simulink model "ev4 (1)"  (R2024a)
settings: Solver=VariableStepAuto  StartTime=0.0  StopTime=601  MaxStep=0.0001  RelTol=1e-3
values from neighbouring files (symbols this model uses):
  a = 1    [evsimcode.m]
  ap = 1.07    [evsimcode.m]
  cd = 0.8    [evsimcode.m]
  ce = 0.9    [evsimcode.m]
  cell_c = 5    [evsimcode.m]
  cell_v = 3.6    [evsimcode.m]
  cr = 0.05    [evsimcode.m]
  cur = data2(:,1)    [evsimcode.m]
  eff = data2(:,5)    [evsimcode.m]
  g = 9.81    [evsimcode.m]
  gr = 9.2    [evsimcode.m]
  lap = 10    [evsimcode.m]
  m = 260    [evsimcode.m]
  me = 0.85    [evsimcode.m]
  ocv = data(:,2)    [evsimcode.m]
  pow = data2(:,2)    [evsimcode.m]
  rho = 1.225    [evsimcode.m]
  rw = 0.2921    [evsimcode.m]
  soc = data(:,1)    [evsimcode.m]
  spd = data2(:,4)    [evsimcode.m]
  te = 0.88    [evsimcode.m]
  theta = 0.6457718232    [evsimcode.m]
  tor = data2(:,2)    [evsimcode.m]
  v = 48    [evsimcode.m]
settings Model: Creator=AXISNIEL  LastModifiedBy=Sai Vivek
settings DebuggingCC: UnconnectedInputMsg=warning  UnconnectedOutputMsg=warning  UnconnectedLineMsg=warning
settings ModelReferenceCC: EnableRefExpFcnMdlSchedulingChecks=on
settings RTWCC: GPUComputeCapability=3.5  DLArmComputeVersion=19.05

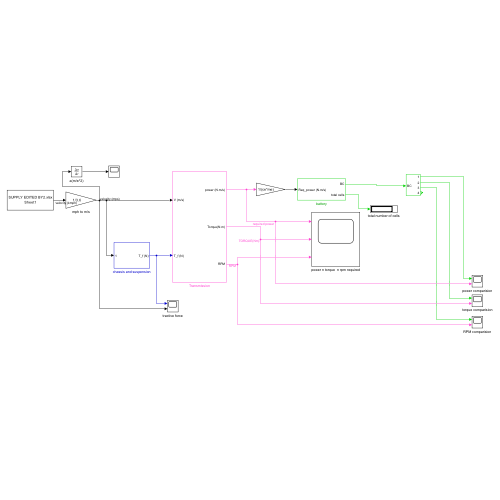
[thumbnail: Simulink's stored preview of the top-level diagram]
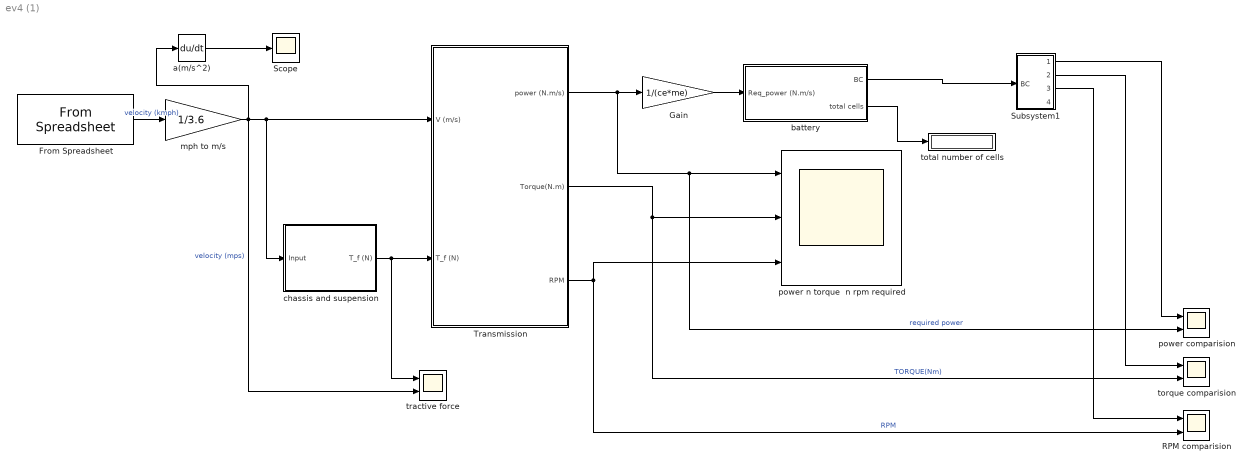
== system ev4 (1) ==
  From Spreadsheet : FromSpreadsheet  FileName=SUPPLY EDITED BY2.xlsx  Range=A1:B601
  Gain : Gain  Gain=1/(ce*me)
  RPM comparision : Scope  NumInputPorts=2
  Scope : Scope
  Subsystem1 : Subsystem
  Transmission : Subsystem
  a(m/s^2) : Derivative
  battery : Subsystem
  chassis and suspension : Subsystem
  mph to m/s : Gain  Gain=1/3.6
  power comparision : Scope  NumInputPorts=2
  power n torque  n rpm required : Scope  NumInputPorts=3
  torque comparision : Scope  NumInputPorts=2
  total number of cells : Display
  tractive force : Scope  NumInputPorts=2
  wires:
  Gain/1 -> battery/1(Req_power (N.m/s))
  Transmission/1(power (N.m/s)) -> Gain/1, power n torque  n rpm required/1, power comparision/2  "required power"
  Transmission/2(Torque(N.m)) -> power n torque  n rpm required/2, torque comparision/2  "TORQUE(Nm)"
  From Spreadsheet/1 -> mph to m/s/1  "velocity (kmph)"
  battery/1(BC) -> Subsystem1/1(BC)
  mph to m/s/1 -> a(m/s^2)/1, chassis and suspension/1(Input), Transmission/1(V (m/s)), tractive force/2  "velocity (mps)"
  Transmission/3(RPM) -> power n torque  n rpm required/3, RPM comparision/2  "RPM"
  chassis and suspension/1(T_f (N)) -> Transmission/2(T_f (N)), tractive force/1
  battery/2(total cells) -> total number of cells/1
  Subsystem1/1(Out1) -> power comparision/1
  Subsystem1/2(Out2) -> torque comparision/1
  Subsystem1/3(Out3) -> RPM comparision/1
  a(m/s^2)/1 -> Scope/1

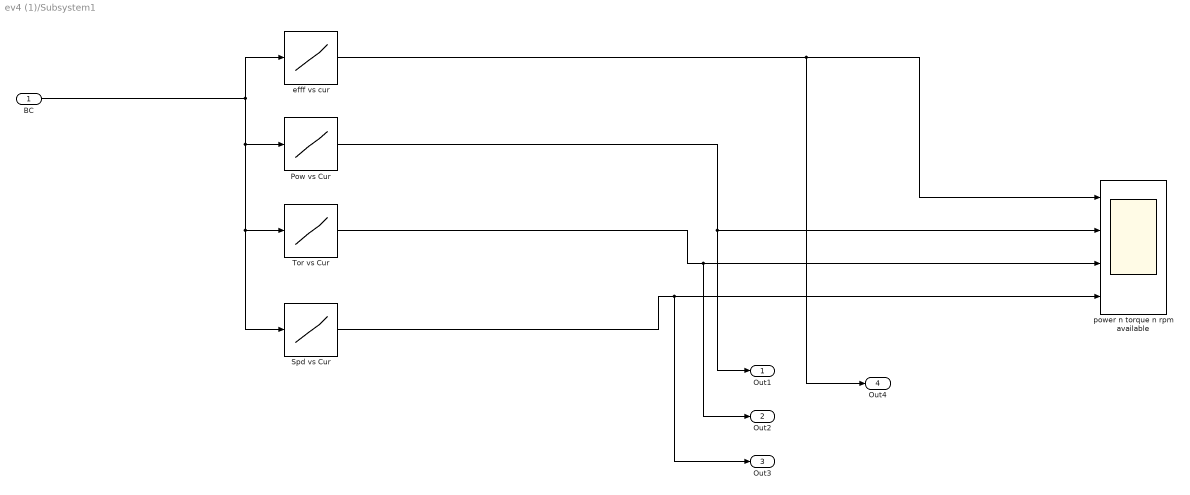
== system ev4 (1)/Subsystem1 ==
  BC : Inport
  Pow vs Cur : Lookup_n-D  NumberOfTableDimensions=1  BreakpointsForDimension1=cur  Table=pow  InternalRulePriority=Speed  RndMeth=Simplest
  Spd vs Cur : Lookup_n-D  NumberOfTableDimensions=1  BreakpointsForDimension1=cur  Table=spd  InternalRulePriority=Speed  RndMeth=Simplest
  Tor vs Cur : Lookup_n-D  NumberOfTableDimensions=1  BreakpointsForDimension1=cur  Table=tor  InternalRulePriority=Speed  RndMeth=Simplest
  efff vs cur : Lookup_n-D  NumberOfTableDimensions=1  BreakpointsForDimension1=cur  Table=eff  InternalRulePriority=Speed  RndMeth=Simplest
  power n torque n rpm available : Scope  NumInputPorts=4
  Out1 : Outport
  Out2 : Outport  Port=2
  Out3 : Outport  Port=3
  Out4 : Outport  Port=4
  wires:
  Spd vs Cur/1 -> Out3/1, power n torque n rpm available/4
  Tor vs Cur/1 -> Out2/1, power n torque n rpm available/3
  Pow vs Cur/1 -> Out1/1, power n torque n rpm available/2
  efff vs cur/1 -> Out4/1, power n torque n rpm available/1
  BC/1 -> Spd vs Cur/1, Tor vs Cur/1, Pow vs Cur/1, efff vs cur/1

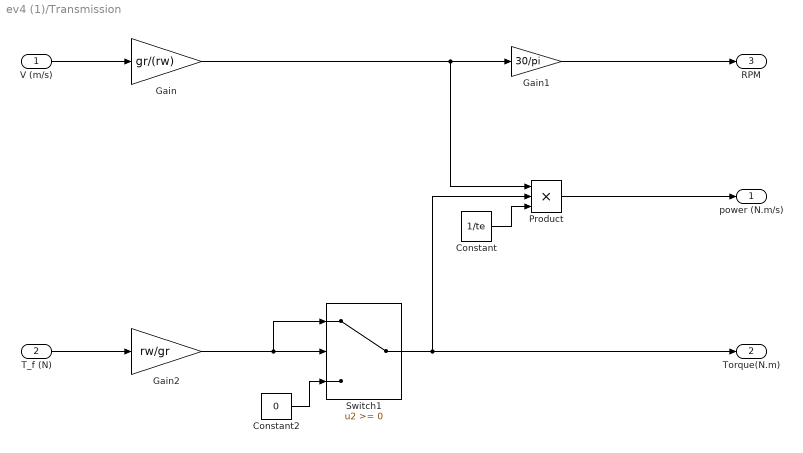
== system ev4 (1)/Transmission ==
  V (m/s) : Inport
  T_f (N) : Inport  Port=2
  Constant : Constant  Value=1/te
  Constant2 : Constant  Value=0
  Gain : Gain  Gain=gr/(rw)
  Gain1 : Gain  Gain=30/pi
  Gain2 : Gain  Gain=rw/gr
  Product : Product  Inputs=3
  Switch1 : Switch  SaturateOnIntegerOverflow=off  InputSameDT=off
  power (N.m/s) : Outport
  Torque(N.m) : Outport  Port=2
  RPM : Outport  Port=3
  wires:
  Gain1/1 -> RPM/1
  V (m/s)/1 -> Gain/1
  Gain/1 -> Product/1, Gain1/1
  T_f (N)/1 -> Gain2/1
  Constant/1 -> Product/3
  Gain2/1 -> Switch1/1, Switch1/2
  Switch1/1 -> Torque(N.m)/1, Product/2
  Constant2/1 -> Switch1/3
  Product/1 -> power (N.m/s)/1

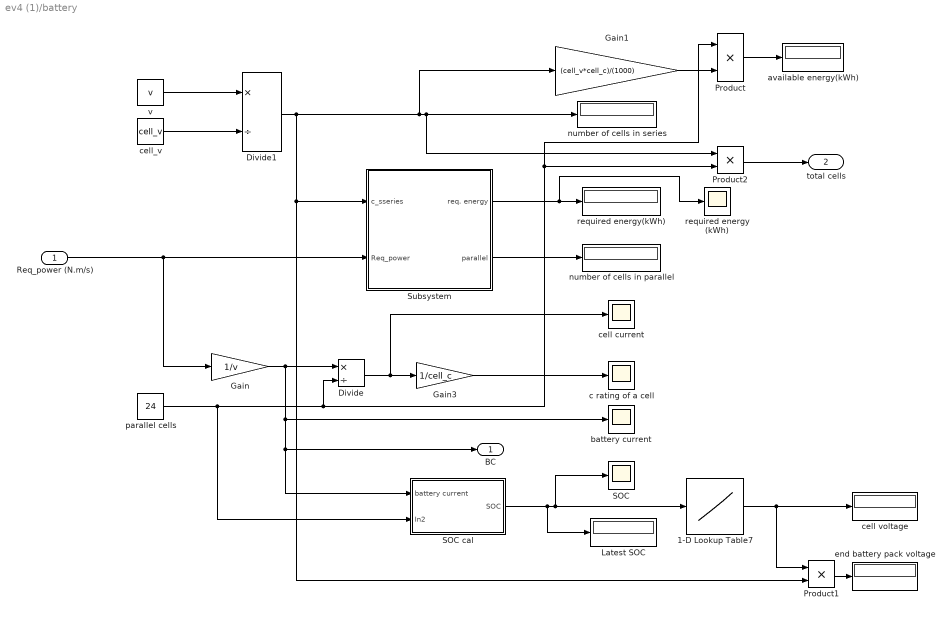
== system ev4 (1)/battery ==
  Req_power (N.m/s) : Inport
  1-D Lookup Table7 : Lookup_n-D  NumberOfTableDimensions=1  BreakpointsForDimension1=soc  Table=ocv  InternalRulePriority=Speed  RndMeth=Simplest
  Divide : Product  Inputs=*/
  Divide1 : Product  Inputs=*/
  Gain : Gain  Gain=1/v
  Gain1 : Gain  Gain=(cell_v*cell_c)/(1000)
  Gain3 : Gain  Gain=1/cell_c
  Latest SOC : Display
  Product : Product
  Product1 : Product
  Product2 : Product
  SOC : Scope
  SOC cal : Subsystem
  Subsystem : Subsystem
  available energy(kWh) : Display
  battery current : Scope
  c rating of a cell : Scope
  cell current : Scope
  cell voltage : Display
  cell_v : Constant  Value=cell_v
  end battery pack voltage : Display
  number of cells in parallel : Display
  number of cells in series : Display
  parallel cells : Constant  Value=24
  required energy (kWh) : Scope
  required energy(kWh) : Display
  v : Constant  Value=v
  BC : Outport
  total cells : Outport  Port=2
  wires:
  1-D Lookup Table7/1 -> Product1/1, cell voltage/1
  Product1/1 -> end battery pack voltage/1
  Subsystem/1(req. energy) -> required energy(kWh)/1, required energy (kWh)/1
  Subsystem/2(parallel) -> number of cells in parallel/1
  Divide1/1 -> Subsystem/1(c_sseries), Product1/2, number of cells in series/1, Product2/1, Gain1/1
  Gain/1 -> SOC cal/1(battery current), BC/1, battery current/1, Divide/1
  Gain3/1 -> c rating of a cell/1
  Divide/1 -> cell current/1, Gain3/1
  SOC cal/1(SOC) -> 1-D Lookup Table7/1, SOC/1, Latest SOC/1
  Product/1 -> available energy(kWh)/1
  Gain1/1 -> Product/2
  Product2/1 -> total cells/1
  cell_v/1 -> Divide1/2
  v/1 -> Divide1/1
  parallel cells/1 -> Divide/2, Product/1, Product2/2, SOC cal/2(In2)
  Req_power (N.m/s)/1 -> Gain/1, Subsystem/2(Req_power)

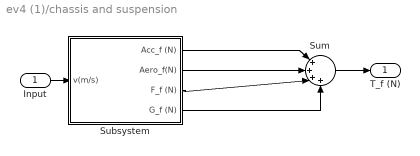
== system ev4 (1)/chassis and suspension ==
  Input : Inport
  Subsystem : Subsystem
  Sum : Sum  Inputs=|++++
  T_f (N) : Outport
  wires:
  Sum/1 -> T_f (N)/1
  Subsystem/1(Acc_f (N)) -> Sum/1
  Subsystem/2(Aero_f(N)) -> Sum/2
  Subsystem/3(F_f (N)) -> Sum/3
  Subsystem/4(G_f (N)) -> Sum/4
  Input/1 -> Subsystem/1(v(m/s))

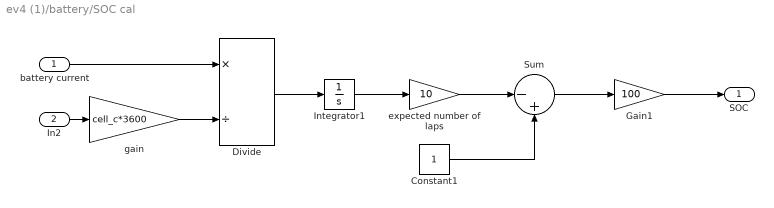
== system ev4 (1)/battery/SOC cal ==
  battery current : Inport
  In2 : Inport  Port=2
  Constant1 : Constant
  Divide : Product  Inputs=*/
  Gain1 : Gain  Gain=100
  Integrator1 : Integrator
  Sum : Sum  Inputs=|-+
  expected number of laps : Gain  Gain=10
  gain : Gain  Gain=cell_c*3600
  SOC : Outport
  wires:
  In2/1 -> gain/1
  gain/1 -> Divide/2
  Divide/1 -> Integrator1/1
  battery current/1 -> Divide/1
  Constant1/1 -> Sum/2
  Sum/1 -> Gain1/1
  Gain1/1 -> SOC/1
  Integrator1/1 -> expected number of laps/1
  expected number of laps/1 -> Sum/1

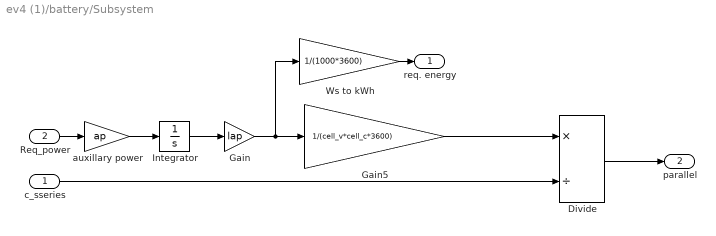
== system ev4 (1)/battery/Subsystem ==
  c_sseries : Inport
  Req_power : Inport  Port=2
  Divide : Product  Inputs=*/
  Gain : Gain  Gain=lap
  Gain5 : Gain  Gain=1/(cell_v*cell_c*3600)
  Integrator : Integrator
  Ws to kWh : Gain  Gain=1/(1000*3600)
  auxillary power : Gain  Gain=ap
  req. energy : Outport
  parallel : Outport  Port=2
  wires:
  Gain5/1 -> Divide/1
  Divide/1 -> parallel/1
  c_sseries/1 -> Divide/2
  Ws to kWh/1 -> req. energy/1
  Integrator/1 -> Gain/1
  Req_power/1 -> auxillary power/1
  auxillary power/1 -> Integrator/1
  Gain/1 -> Ws to kWh/1, Gain5/1

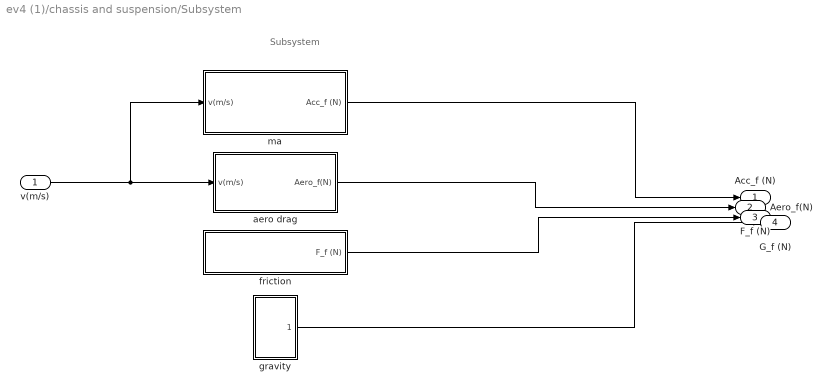
== system ev4 (1)/chassis and suspension/Subsystem ==
  note: Subsystem
  v(m/s) : Inport
  aero drag : Subsystem
  friction : Subsystem
  gravity : Subsystem
  ma : Subsystem
  Acc_f (N) : Outport
  Aero_f(N) : Outport  Port=2
  F_f (N) : Outport  Port=3
  G_f (N) : Outport  Port=4
  wires:
  v(m/s)/1 -> ma/1(v(m/s)), aero drag/1(v(m/s))
  friction/1(F_f (N)) -> F_f (N)/1
  gravity/1(G_f (N)) -> G_f (N)/1
  ma/1(Acc_f (N)) -> Acc_f (N)/1
  aero drag/1(Aero_f(N)) -> Aero_f(N)/1

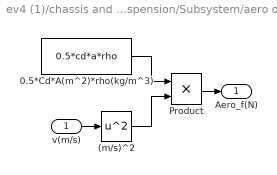
== system ev4 (1)/chassis and suspension/Subsystem/aero drag ==
  v(m/s) : Inport
  (m/s)^2 : Math  Operator=square
  0.5*Cd*A(m^2)*rho(kg/m^3) : Constant  Value=0.5*cd*a*rho
  Product : Product
  Aero_f(N) : Outport
  wires:
  0.5*Cd*A(m^2)*rho(kg/m^3)/1 -> Product/1
  (m/s)^2/1 -> Product/2
  Product/1 -> Aero_f(N)/1
  v(m/s)/1 -> (m/s)^2/1

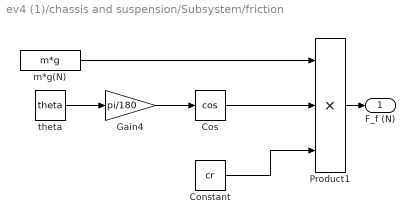
== system ev4 (1)/chassis and suspension/Subsystem/friction ==
  Constant : Constant  Value=cr
  Cos : Trigonometry  Operator=cos
  Gain4 : Gain  Gain=pi/180
  Product1 : Product  Inputs=3
  m*g(N) : Constant  Value=m*g
  theta : Constant  Value=theta
  F_f (N) : Outport
  wires:
  Gain4/1 -> Cos/1
  theta/1 -> Gain4/1
  Cos/1 -> Product1/2
  m*g(N)/1 -> Product1/1
  Constant/1 -> Product1/3
  Product1/1 -> F_f (N)/1

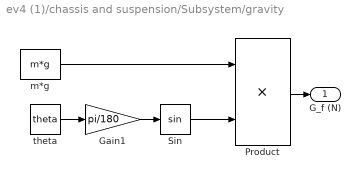
== system ev4 (1)/chassis and suspension/Subsystem/gravity ==
  Gain1 : Gain  Gain=pi/180
  Product : Product
  Sin : Trigonometry
  m*g : Constant  Value=m*g
  theta : Constant  Value=theta
  G_f (N) : Outport
  wires:
  theta/1 -> Gain1/1
  Sin/1 -> Product/2
  Gain1/1 -> Sin/1
  m*g/1 -> Product/1
  Product/1 -> G_f (N)/1

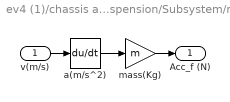
== system ev4 (1)/chassis and suspension/Subsystem/ma ==
  v(m/s) : Inport
  a(m/s^2) : Derivative
  mass(Kg) : Gain  Gain=m
  Acc_f (N) : Outport
  wires:
  mass(Kg)/1 -> Acc_f (N)/1
  a(m/s^2)/1 -> mass(Kg)/1
  v(m/s)/1 -> a(m/s^2)/1
